simulink model "ARDroneHover_2020b"  (R2020b)
settings: Solver=ode1  StartTime=0.0  StopTime=inf  FixedStep=sampleTime  RelTol=1e-3  EnableMultiTasking=on
values from neighbouring files (symbols this model uses):
  sampleTime = 0.01    [setupHover.m]    (also in setupTT.m; setupWPTracking.m)
undefined symbols (not defined in the file or in its folder): DiscIntNeverNeededParam, Standard_Devices, UDP_Protocol
libraries: hdlsllib x6, dspnetwork x4, sldrtlib x3, simulink x1
(part 1 of 2)
settings Model: EnablePacing=on  ExtModeTrigDuration=100000  Creator=Paul  LastModifiedBy=dsor
settings SolverCC: AutoInsertRateTranBlk=on
settings DataIOCC: LimitDataPoints=on  SaveFormat=StructureWithTime  SignalLoggingSaveFormat=ModelDataLogs  ReturnWorkspaceOutputs=off  TimeSaveName=time
settings OptimizationCC: BlockReduction=off  OptimizeBlockIOStorage=off  BufferReuse=off  GlobalBufferReuse=off  ExpressionFolding=off  ExpressionDepthLimit=2147483647  LocalBlockOutputs=off  InitFltsAndDblsToZero=on  OptimizeDataStoreBuffers=off  BusAssignmentInplaceUpdate=off
settings DebuggingCC: UnderspecifiedInitializationDetection=Classic  MergeDetectMultiDrivingBlocksExec=none  SolverPrmCheckMsg=warning  FcnCallInpInsideContextMsg=warning  StateNameClashWarn=warning  SFUnexpectedBacktrackingDiag=warning  SFNoUnconditionalDefaultTransitionDiag=warning  SFExecutionAtInitializationDiag=none  ArithmeticOperatorsInVariantConditions=warning
settings ModelReferenceCC: PropagateSignalLabelsOutOfModel=off
settings SFSimCC: SimUseLocalCustomCode=off  CustomCodeUndefinedFunction=UseInterfaceOnly
settings RTWCC: Description=Simulink Desktop Real-Time  SystemTargetFile=sldrt.tlc  TemplateMakefile=sldrt.tmf  RTWUseLocalCustomCode=off  RTWCompilerOptimization=on
settings CodeAppCC: MaxIdLength=95  StateflowObjectComments=on
settings SimulinkDesktopRealTimeCC: TargetPreCompLibLocation=C:\Program Files\Polyspace\R2020b\toolbox\sldrt\lib\win64  TargetLangStandard=C89/C90 (ANSI)
settings ConfigComp: CovMetricSettings=dw  CovSaveCumulativeToWorkspaceVar=on  CovSaveSingleToWorkspaceVar=on  CovExternalEMLEnable=off

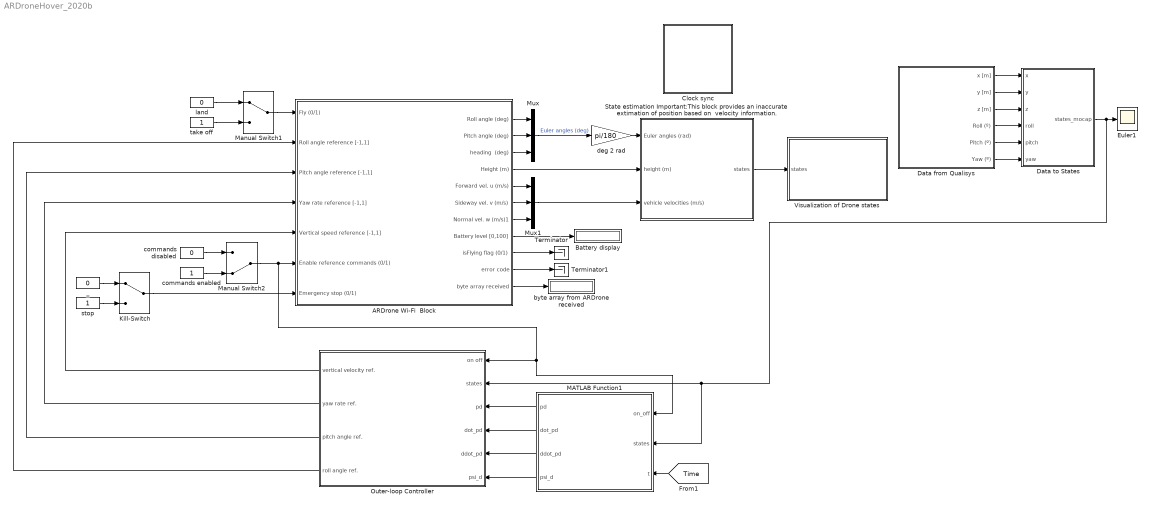
== system ARDroneHover_2020b ==
  ARDrone Wi-Fi  Block : Subsystem  AncestorBlock="ARBlocks/ARDrone Wi-Fi  Block"
  Battery display : Display
  Clock sync : Subsystem
  Data from Qualisys : Subsystem
  Data to States : Subsystem
  Euler1 : Scope
  Kill-Switch : ManualSwitch
  MATLAB Function1 : MATLAB Function  TreatAsAtomicUnit=on  SystemSampleTime=sampleTime
  Manual Switch1 : ManualSwitch
  Manual Switch2 : ManualSwitch  CurrentSetting=0
  Mux : Mux  Inputs=3
  Mux1 : Mux  Inputs=3
  Outer-loop Controller : Subsystem
  "State estimation Important:This block provides an inaccurate extimation of position based on  velocity information. " : Subsystem  AncestorBlock=|
      | ARBlocks/Position estimation
      | Important:This block provides an 
      | inaccurate extimation of position 
      | based on  velocity information.
  Terminator : Terminator
  Terminator1 : Terminator
  Visualization of Drone states : Subsystem
  _ : Constant  Value=0
  "byte array from ARDrone received " : Display
  commands disabled : Constant  Value=0
  commands enabled : Constant
  deg 2 rad : Gain  Gain=pi/180
  land : Constant  Value=0
  stop : Constant
  take off : Constant
  wires:
  _/1 -> Kill-Switch/1
  stop/1 -> Kill-Switch/2
  land/1 -> Manual Switch1/1
  take off/1 -> Manual Switch1/2
  commands disabled/1 -> Manual Switch2/1
  commands enabled/1 -> Manual Switch2/2
  Manual Switch1/1 -> ARDrone Wi-Fi  Block/1(Fly (0/1))
  Manual Switch2/1 -> ARDrone Wi-Fi  Block/6(Enable reference commands (0/1)), MATLAB Function1/1(on_off), Outer-loop Controller/1(on off)
  Kill-Switch/1 -> ARDrone Wi-Fi  Block/7(Emergency stop (0/1))
  ARDrone Wi-Fi  Block/1(Roll angle (deg)) -> Mux/1
  ARDrone Wi-Fi  Block/2(Pitch angle (deg)) -> Mux/2
  ARDrone Wi-Fi  Block/5(Forward vel. u (m/s)) -> Mux1/1
  ARDrone Wi-Fi  Block/6(Sideway vel. v (m/s)) -> Mux1/2
  ARDrone Wi-Fi  Block/7(Normal vel. w (m/s)1) -> Mux1/3
  Mux/1 -> deg 2 rad/1  "Euler angles (deg)"
  ARDrone Wi-Fi  Block/8(Battery level [0,100]) -> Battery display/1
  Outer-loop Controller/1(vertical velocity ref.) -> ARDrone Wi-Fi  Block/5(Vertical speed reference [-1,1])
  "State estimation Important:This block provides an inaccurate extimation of position based on  velocity information. "/1(states) -> Visualization of Drone states/1(states)
  deg 2 rad/1 -> "State estimation Important:This block provides an inaccurate extimation of position based on  velocity information. "/1(Euler angles (rad))
  Mux1/1 -> "State estimation Important:This block provides an inaccurate extimation of position based on  velocity information. "/3(vehicle velocities (m/s))
  ARDrone Wi-Fi  Block/3(heading  (deg)) -> Mux/3
  ARDrone Wi-Fi  Block/9(isFlying flag (0/1)) -> Terminator/1
  ARDrone Wi-Fi  Block/10(error code) -> Terminator1/1
  ARDrone Wi-Fi  Block/11(byte array received) -> "byte array from ARDrone received "/1
  Outer-loop Controller/2(yaw rate ref.) -> ARDrone Wi-Fi  Block/4(Yaw rate reference [-1,1])
  MATLAB Function1/2(dot_pd) -> Outer-loop Controller/4(dot_pd)
  MATLAB Function1/3(ddot_pd) -> Outer-loop Controller/5(ddot_pd)
  MATLAB Function1/4(psi_d) -> Outer-loop Controller/6(psi_d)
  MATLAB Function1/1(pd) -> Outer-loop Controller/3(pd)
  Data from Qualisys/1(x [m]) -> Data to States/1(x)
  Data from Qualisys/2(y [m]) -> Data to States/2(y)
  Data from Qualisys/3(z [m]) -> Data to States/3(z)
  Data from Qualisys/4(Roll (º)) -> Data to States/4(roll)
  Data from Qualisys/5(Pitch (º)) -> Data to States/5(pitch)
  Data from Qualisys/6(Yaw (º)) -> Data to States/6(yaw)
  [Time] -> MATLAB Function1/3(t)
  ARDrone Wi-Fi  Block/4(Height (m)) -> "State estimation Important:This block provides an inaccurate extimation of position based on  velocity information. "/2(height (m))
  Data to States/1(states_mocap) -> MATLAB Function1/2(states), Outer-loop Controller/2(states), Euler1/1
  Outer-loop Controller/4(roll angle ref.) -> ARDrone Wi-Fi  Block/2(Roll angle reference [-1,1])
  Outer-loop Controller/3(pitch angle ref.) -> ARDrone Wi-Fi  Block/3(Pitch angle reference [-1,1])

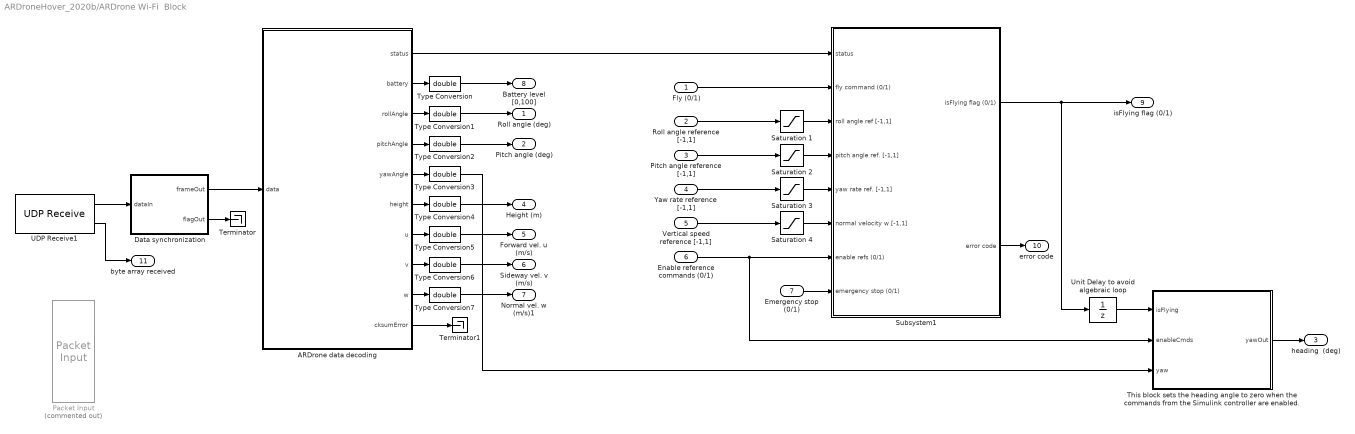
== system ARDroneHover_2020b/ARDrone Wi-Fi  Block ==
  Fly (0/1) : Inport
  Roll angle reference [-1,1] : Inport  Port=2
  Pitch angle reference [-1,1] : Inport  Port=3
  Yaw rate reference [-1,1] : Inport  Port=4
  Vertical speed reference [-1,1] : Inport  Port=5
  Enable reference commands (0/1) : Inport  Port=6
  Emergency stop (0/1) : Inport  Port=7
  ARDrone data decoding : MATLAB Function  TreatAsAtomicUnit=on
  "Data synchronization " : MATLAB Function  TreatAsAtomicUnit=on
  Packet Input : sldrtlib/Packet Input  Commented=on  SampleTime=sampleTime  MaxMissedTicks=100  ShowMissedTicks=off  YieldWhenWaiting=off  DrvName=Standard_Devices/UDP_Protocol  DrvAddress=5554  DrvOptions=[3232235777 5554]  PacketSize=500  DataTypes='500*uint8'  ShowReady=on  ShowError=off  PacketID=1  ByteOrder=1  ShowTimestamp=off
      settings: AttributesFormatString=UDP Protocol [5554]
  Saturation {1..4} (4 alike) : Saturate  UpperLimit=1  LowerLimit=-1
  Subsystem1 : Subsystem
  Terminator : Terminator
  Terminator1 : Terminator
  "This block sets the heading angle to zero when the commands from the Simulink controller are enabled. " : MATLAB Function  TreatAsAtomicUnit=on
  Type Conversion{,1..7} (8 alike) : DataTypeConversion  OutDataTypeStr=double
  UDP Receive1 : dspnetwork/UDP Receive  localURL='0.0.0.0'  localPort=5554  remoteURL='192.168.1.1'  remotePort=-1  recvBufferSize=500  dims=500  signalDatatype=uint8  isComplex=off  isVarSize=off  showBlockingTime=off  blockingTime=0  sampletime=sampleTime  blockPlatform=[]
  Unit Delay to avoid algebraic loop : UnitDelay  SampleTime=-1  HasFrameUpgradeWarning=on
  Roll angle (deg) : Outport  VectorParamsAs1DForOutWhenUnconnected=off
  Pitch angle (deg) : Outport  Port=2  VectorParamsAs1DForOutWhenUnconnected=off
  heading  (deg) : Outport  Port=3  VectorParamsAs1DForOutWhenUnconnected=off
  Height (m) : Outport  Port=4  VectorParamsAs1DForOutWhenUnconnected=off
  Forward vel. u (m/s) : Outport  Port=5  VectorParamsAs1DForOutWhenUnconnected=off
  Sideway vel. v (m/s) : Outport  Port=6  VectorParamsAs1DForOutWhenUnconnected=off
  Normal vel. w (m/s)1 : Outport  Port=7  VectorParamsAs1DForOutWhenUnconnected=off
  Battery level [0,100] : Outport  Port=8  VectorParamsAs1DForOutWhenUnconnected=off
  isFlying flag (0/1) : Outport  Port=9  VectorParamsAs1DForOutWhenUnconnected=off
  error code : Outport  Port=10  VectorParamsAs1DForOutWhenUnconnected=off
  byte array received : Outport  Port=11  VectorParamsAs1DForOutWhenUnconnected=off
  wires:
  Unit Delay to avoid algebraic loop/1 -> "This block sets the heading angle to zero when the commands from the Simulink controller are enabled. "/1(isFlying)
  "Data synchronization "/2(flagOut) -> Terminator/1
  Saturation 4/1 -> Subsystem1/6(normal velocity w [-1,1])
  Saturation 3/1 -> Subsystem1/5(yaw rate ref. [-1,1])
  Saturation 2/1 -> Subsystem1/4(pitch angle ref. [-1,1])
  Saturation 1/1 -> Subsystem1/3(roll angle ref [-1,1])
  Fly (0/1)/1 -> Subsystem1/2(fly command (0/1))
  "This block sets the heading angle to zero when the commands from the Simulink controller are enabled. "/1(yawOut) -> heading  (deg)/1
  Type Conversion3/1 -> "This block sets the heading angle to zero when the commands from the Simulink controller are enabled. "/3(yaw)
  Type Conversion7/1 -> Normal vel. w (m/s)1/1
  Type Conversion6/1 -> Sideway vel. v (m/s)/1
  Type Conversion5/1 -> Forward vel. u (m/s)/1
  Type Conversion4/1 -> Height (m)/1
  Type Conversion2/1 -> Pitch angle (deg)/1
  Type Conversion1/1 -> Roll angle (deg)/1
  Type Conversion/1 -> Battery level [0,100]/1
  ARDrone data decoding/10(cksumError) -> Terminator1/1
  Subsystem1/2(error code) -> error code/1
  Subsystem1/1(isFlying flag (0/1)) -> isFlying flag (0/1)/1, Unit Delay to avoid algebraic loop/1
  Emergency stop (0/1)/1 -> Subsystem1/8(emergency stop (0/1))
  Enable reference commands (0/1)/1 -> Subsystem1/7(enable refs (0/1)), "This block sets the heading angle to zero when the commands from the Simulink controller are enabled. "/2(enableCmds)
  Vertical speed reference [-1,1]/1 -> Saturation 4/1
  Yaw rate reference [-1,1]/1 -> Saturation 3/1
  Pitch angle reference [-1,1]/1 -> Saturation 2/1
  Roll angle reference [-1,1]/1 -> Saturation 1/1
  ARDrone data decoding/1(status) -> Subsystem1/1(status)
  UDP Receive1/2 -> byte array received/1
  ARDrone data decoding/9(w) -> Type Conversion7/1
  ARDrone data decoding/8(v) -> Type Conversion6/1
  ARDrone data decoding/7(u) -> Type Conversion5/1
  ARDrone data decoding/4(pitchAngle) -> Type Conversion2/1
  ARDrone data decoding/3(rollAngle) -> Type Conversion1/1
  ARDrone data decoding/6(height) -> Type Conversion4/1
  ARDrone data decoding/2(battery) -> Type Conversion/1
  ARDrone data decoding/5(yawAngle) -> Type Conversion3/1
  "Data synchronization "/1(frameOut) -> ARDrone data decoding/1(data)
  UDP Receive1/1 -> "Data synchronization "/1(dataIn)

== system ARDroneHover_2020b/Clock sync ==
  Clock1 : Clock
  To Workspace6 : ToWorkspace  VariableName=timeRT  SampleTime=sampleTime
  tag scope: Time=global
  wires:
  Clock1/1 -> [Time], To Workspace6/1

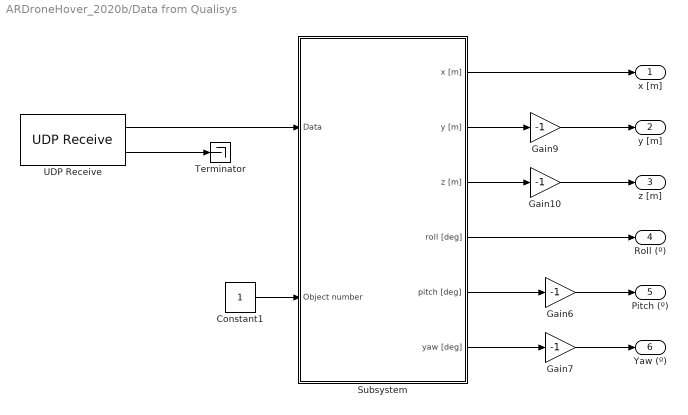
== system ARDroneHover_2020b/Data from Qualisys ==
  Constant1 : Constant
  Gain{6..7,9..10} (4 alike) : Gain  Gain=-1
  Subsystem : Subsystem
  Terminator : Terminator
  UDP Receive : dspnetwork/UDP Receive  localURL='0.0.0.0'  localPort=9089  remoteURL='169.254.54.40'  remotePort=-1  recvBufferSize=64  dims=255  signalDatatype=uint8  isComplex=off  isVarSize=off  showBlockingTime=off  blockingTime=0  sampletime=sampleTime  blockPlatform=[]
  x [m] : Outport
  y [m] : Outport  Port=2
  z [m] : Outport  Port=3
  Roll (º) : Outport  Port=4
  Pitch (º) : Outport  Port=5
  Yaw (º) : Outport  Port=6
  wires:
  Subsystem/3(z [m]) -> Gain10/1
  Subsystem/2(y [m]) -> Gain9/1
  Constant1/1 -> Subsystem/2(Object number)
  Subsystem/5(pitch [deg]) -> Gain6/1
  Gain7/1 -> Yaw (º)/1
  Gain10/1 -> z [m]/1
  Gain6/1 -> Pitch (º)/1
  Gain9/1 -> y [m]/1
  Subsystem/1(x [m]) -> x [m]/1
  UDP Receive/2 -> Terminator/1
  UDP Receive/1 -> Subsystem/1(Data)
  Subsystem/4(roll [deg]) -> Roll (º)/1
  Subsystem/6(yaw [deg]) -> Gain7/1

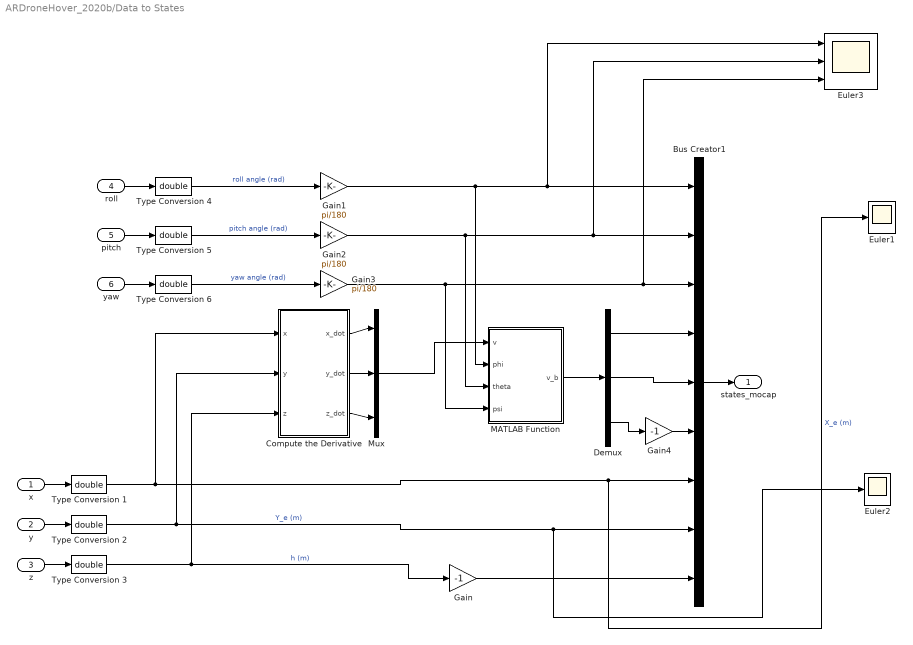
== system ARDroneHover_2020b/Data to States ==
  x : Inport
  y : Inport  Port=2
  z : Inport  Port=3
  roll : Inport  Port=4
  pitch : Inport  Port=5
  yaw : Inport  Port=6
  Bus Creator1 : BusCreator  Inputs=9
  Compute the Derivative : Subsystem
  Demux : Demux  Outputs=3
  Euler1 : Scope
  Euler2 : Scope
  Euler3 : Scope  NumInputPorts=3
  Gain : Gain  Gain=-1
  Gain1 : Gain  Gain=pi/180
  Gain2 : Gain  Gain=pi/180
  Gain3 : Gain  Gain=pi/180
  Gain4 : Gain  Gain=-1
  MATLAB Function : MATLAB Function  TreatAsAtomicUnit=on
  Mux : Mux  Inputs=3
  Type Conversion {1..6} (6 alike) : DataTypeConversion  OutDataTypeStr=double
  states_mocap : Outport  VectorParamsAs1DForOutWhenUnconnected=off
  wires:
  x/1 -> Type Conversion 1/1
  y/1 -> Type Conversion 2/1
  z/1 -> Type Conversion 3/1
  roll/1 -> Type Conversion 4/1
  pitch/1 -> Type Conversion 5/1
  yaw/1 -> Type Conversion 6/1
  Type Conversion 6/1 -> Gain3/1  "yaw angle (rad)"
  Type Conversion 4/1 -> Gain1/1  "roll angle (rad)"
  Type Conversion 5/1 -> Gain2/1  "pitch angle (rad)"
  Type Conversion 1/1 -> Compute the Derivative/1(x), Euler1/1, Bus Creator1/7  "X_e (m)"
  Type Conversion 3/1 -> Compute the Derivative/3(z), Gain/1  "h (m)"
  Type Conversion 2/1 -> Compute the Derivative/2(y), Euler2/1, Bus Creator1/8  "Y_e (m)"
  Gain/1 -> Bus Creator1/9
  Compute the Derivative/1(x_dot) -> Mux/1
  Compute the Derivative/2(y_dot) -> Mux/2
  Compute the Derivative/3(z_dot) -> Mux/3
  MATLAB Function/1(v_b) -> Demux/1
  Mux/1 -> MATLAB Function/1(v)
  Gain1/1 -> Euler3/1, Bus Creator1/1, MATLAB Function/2(phi)
  Gain2/1 -> MATLAB Function/3(theta), Euler3/2, Bus Creator1/2
  Gain3/1 -> MATLAB Function/4(psi), Euler3/3, Bus Creator1/3
  Demux/1 -> Bus Creator1/4
  Demux/2 -> Bus Creator1/5
  Gain4/1 -> Bus Creator1/6
  Demux/3 -> Gain4/1
  Bus Creator1/1 -> states_mocap/1

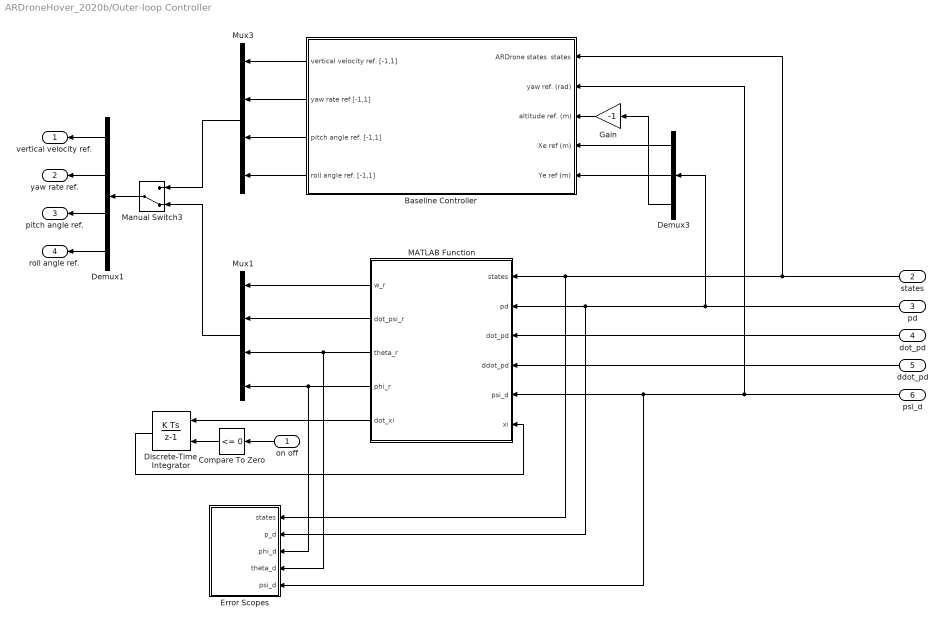
== system ARDroneHover_2020b/Outer-loop Controller ==
  on off : Inport  PortDimensions=1
  states : Inport  Port=2
  pd : Inport  Port=3  PortDimensions=[3 1]
  dot_pd : Inport  Port=4  PortDimensions=[3 1]
  ddot_pd : Inport  Port=5  PortDimensions=[3 1]
  psi_d : Inport  Port=6  PortDimensions=1
  Baseline Controller : Subsystem  AncestorBlock=ARBlocks/Baseline Controller
  Compare To Zero : simulink/Logic and Bit Operations/Compare To Zero  relop=<=  OutDataTypeStr=boolean
  Demux1 : Demux  Outputs=[1,1,1,1]
  Demux3 : Demux  Outputs=[1,1,1]
  Discrete-Time Integrator : DiscreteIntegrator  ExternalReset=level  InitialCondition=[0;0;0;0]  SampleTime=sampleTime  LimitOutput=on  UpperSaturationLimit=100  LowerSaturationLimit=-100  ICPrevOutput=DiscIntNeverNeededParam  ICPrevScaledInput=DiscIntNeverNeededParam
  Error Scopes : Subsystem
  Gain : Gain  Gain=-1
  MATLAB Function : MATLAB Function  TreatAsAtomicUnit=on  SystemSampleTime=sampleTime
  Manual Switch3 : ManualSwitch  CurrentSetting=0
  Mux1 : Mux  Inputs=[1,1,1,1]
  Mux3 : Mux  Inputs=[1,1,1,1]
  vertical velocity ref. : Outport  VectorParamsAs1DForOutWhenUnconnected=off
  yaw rate ref. : Outport  Port=2  VectorParamsAs1DForOutWhenUnconnected=off
  pitch angle ref. : Outport  Port=3  VectorParamsAs1DForOutWhenUnconnected=off
  roll angle ref. : Outport  Port=4  VectorParamsAs1DForOutWhenUnconnected=off
  wires:
  states/1 -> MATLAB Function/1(states), Error Scopes/1(states), Baseline Controller/1("ARDrone states  states ")
  MATLAB Function/1(w_r) -> Mux1/1
  MATLAB Function/3(theta_r) -> Error Scopes/4(theta_d), Mux1/3
  MATLAB Function/4(phi_r) -> Mux1/4, Error Scopes/3(phi_d)
  MATLAB Function/2(dot_psi_r) -> Mux1/2
  MATLAB Function/5(dot_xi) -> Discrete-Time Integrator/1
  Discrete-Time Integrator/1 -> MATLAB Function/6(xi)
  pd/1 -> Demux3/1, MATLAB Function/2(pd), Error Scopes/2(p_d)
  dot_pd/1 -> MATLAB Function/3(dot_pd)
  ddot_pd/1 -> MATLAB Function/4(ddot_pd)
  psi_d/1 -> Baseline Controller/2(yaw ref. (rad)), MATLAB Function/5(psi_d), Error Scopes/5(psi_d)
  Demux3/1 -> Baseline Controller/4(Xe ref (m))
  Demux3/2 -> Baseline Controller/5(Ye ref (m))
  Demux3/3 -> Gain/1
  Baseline Controller/4(roll angle ref. [-1,1]) -> Mux3/4
  Baseline Controller/3(pitch angle ref. [-1,1]) -> Mux3/3
  Baseline Controller/2(yaw rate ref [-1,1]) -> Mux3/2
  Baseline Controller/1(vertical velocity ref. [-1,1]) -> Mux3/1
  Mux3/1 -> Manual Switch3/1
  Demux1/1 -> vertical velocity ref./1
  Demux1/2 -> yaw rate ref./1
  Demux1/3 -> pitch angle ref./1
  Demux1/4 -> roll angle ref./1
  Manual Switch3/1 -> Demux1/1
  Mux1/1 -> Manual Switch3/2
  on off/1 -> Compare To Zero/1
  Compare To Zero/1 -> Discrete-Time Integrator/2
  Gain/1 -> Baseline Controller/3(altitude ref. (m))

== system ARDroneHover_2020b/State estimation Important:This block provides an inaccurate extimation of position based on  velocity information.  ==
  Euler angles (rad) : Inport
  height (m) : Inport  Port=2
  vehicle velocities (m/s) : Inport  Port=3
  Bus Creator1 : BusCreator  Inputs=9
  Demux : Demux  Outputs=3
  Demux1 : Demux  Outputs=3
  Demux2 : Demux  Outputs=3
  Position estimation : Subsystem
  states : Outport  VectorParamsAs1DForOutWhenUnconnected=off
  wires:
  height (m)/1 -> Position estimation/2(height (m))
  Bus Creator1/1 -> states/1
  Demux2/3 -> Bus Creator1/9  "h (m)"
  Demux2/2 -> Bus Creator1/8  "Y_e (m)"
  Demux2/1 -> Bus Creator1/7  "X_e (m)"
  Demux1/3 -> Bus Creator1/6  "vertical velocity - h_dot (m/s)"
  Demux1/2 -> Bus Creator1/5  "sideward velocity - v (m/s)"
  Demux1/1 -> Bus Creator1/4  "forward velocity- u (m/s)"
  Demux/3 -> Bus Creator1/3  "yaw angle (rad)"
  Demux/2 -> Bus Creator1/2  "pitch angle (rad)"
  Demux/1 -> Bus Creator1/1  "roll angle (rad)"
  Position estimation/1(Inertial position Xe,Ye,h (m)) -> Demux2/1
  Euler angles (rad)/1 -> Demux/1, Position estimation/1(Vehicle euler angles (rad))
  vehicle velocities (m/s)/1 -> Position estimation/3(vehicle frame velocities (m/s)), Demux1/1

== system ARDroneHover_2020b/Visualization of Drone states ==
  states : Inport
  Bus Selector2 : BusSelector  OutputSignals=yaw angle (rad),X_e (m),Y_e (m),h (m)
  Height (m) : Scope
  Inertial position along Xe (m) : Scope
  Inertial position along Ye (m) : Scope
  To Workspace : ToWorkspace  VariableName=states  SaveFormat=Structure With Time  SampleTime=-1
  deg 2 rad1 : Gain  Gain=180/pi
  heading (deg) : Scope
  wires:
  states/1 -> To Workspace/1, Bus Selector2/1
  Bus Selector2/1 -> deg 2 rad1/1  "<yaw angle (rad)>"
  Bus Selector2/2 -> Inertial position along Xe (m)/1  "<X_e (m)>"
  Bus Selector2/3 -> Inertial position along Ye (m)/1  "<Y_e (m)>"
  Bus Selector2/4 -> Height (m)/1  "<h (m)>"
  deg 2 rad1/1 -> heading (deg)/1

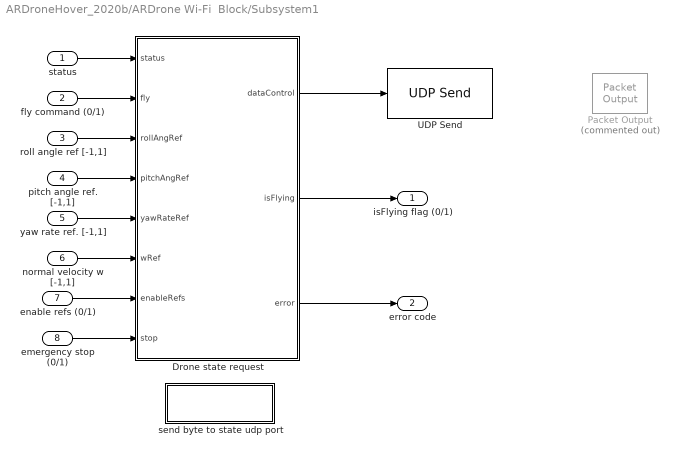
== system ARDroneHover_2020b/ARDrone Wi-Fi  Block/Subsystem1 ==
  status : Inport
  fly command (0/1) : Inport  Port=2
  roll angle ref [-1,1] : Inport  Port=3
  pitch angle ref. [-1,1] : Inport  Port=4
  yaw rate ref. [-1,1] : Inport  Port=5
  normal velocity w [-1,1] : Inport  Port=6
  enable refs (0/1) : Inport  Port=7
  emergency stop (0/1) : Inport  Port=8
  Drone state request : MATLAB Function  TreatAsAtomicUnit=on  SystemSampleTime=sampleTime
  Packet Output : sldrtlib/Packet Output  Commented=on  SampleTime=sampleTime*7  MaxMissedTicks=100  ShowMissedTicks=off  YieldWhenWaiting=off  DrvName=Standard_Devices/UDP_Protocol  DrvAddress=5556  DrvOptions=[3232235777 5556]  PacketSize=150  DataTypes='150*uint8'  ShowReady=off  ShowError=off  PacketID=1  ByteOrder=1  InitialValue=[]  FinalValue=[]
      settings: AttributesFormatString=UDP Protocol [5556]
  UDP Send : dspnetwork/UDP Send  remoteURL='192.168.1.1'  remotePort=5556  localURL='0.0.0.0'  localPortSource=Specify via dialog  localPort=5556  sendBufferSize=8192  sampletime=-1  blockPlatform=[]  separateLengthPort=0
  "send byte to state udp port " : Subsystem
  isFlying flag (0/1) : Outport  VectorParamsAs1DForOutWhenUnconnected=off
  error code : Outport  Port=2  VectorParamsAs1DForOutWhenUnconnected=off
  wires:
  Drone state request/3(error) -> error code/1
  emergency stop (0/1)/1 -> Drone state request/8(stop)
  enable refs (0/1)/1 -> Drone state request/7(enableRefs)
  normal velocity w [-1,1]/1 -> Drone state request/6(wRef)
  yaw rate ref. [-1,1]/1 -> Drone state request/5(yawRateRef)
  roll angle ref [-1,1]/1 -> Drone state request/3(rollAngRef)
  Drone state request/2(isFlying) -> isFlying flag (0/1)/1
  status/1 -> Drone state request/1(status)
  pitch angle ref. [-1,1]/1 -> Drone state request/4(pitchAngRef)
  fly command (0/1)/1 -> Drone state request/2(fly)
  Drone state request/1(dataControl) -> UDP Send/1

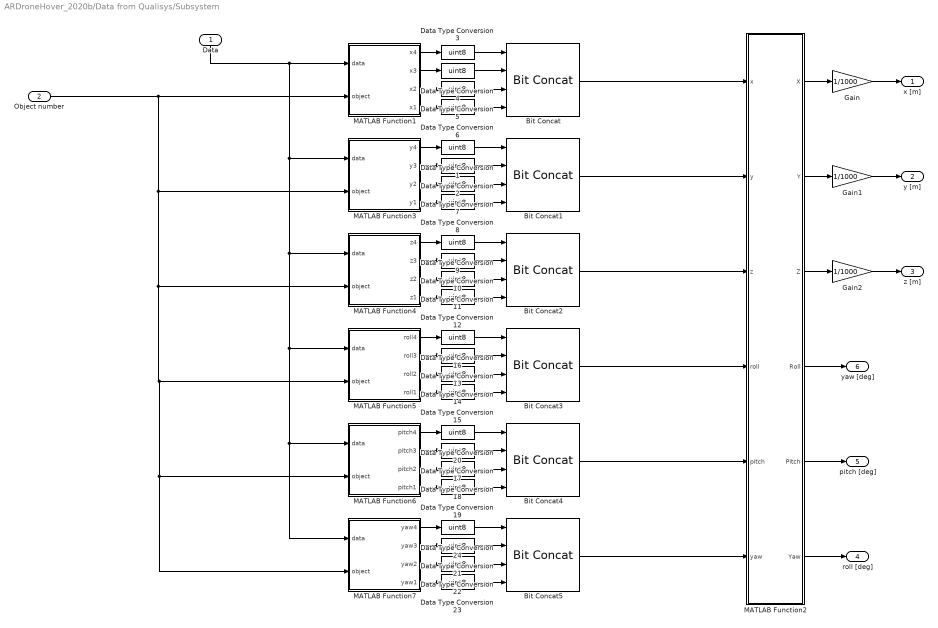
== system ARDroneHover_2020b/Data from Qualisys/Subsystem ==
  Data : Inport
  Object number : Inport  Port=2
  Bit Concat{,1..5} (6 alike) : hdlsllib/Logic and Bit Operations/Bit Concat  numInputs=4
  Data Type Conversion{1..24} (24 alike) : DataTypeConversion  OutDataTypeStr=uint8
  Gain : Gain  Gain=1/1000
  Gain1 : Gain  Gain=1/1000
  Gain2 : Gain  Gain=1/1000
  MATLAB Function1 : MATLAB Function  TreatAsAtomicUnit=on
  MATLAB Function2 : MATLAB Function  TreatAsAtomicUnit=on
  MATLAB Function3 : MATLAB Function  TreatAsAtomicUnit=on
  MATLAB Function4 : MATLAB Function  TreatAsAtomicUnit=on
  MATLAB Function5 : MATLAB Function  TreatAsAtomicUnit=on
  MATLAB Function6 : MATLAB Function  TreatAsAtomicUnit=on
  MATLAB Function7 : MATLAB Function  TreatAsAtomicUnit=on
  x [m] : Outport  VectorParamsAs1DForOutWhenUnconnected=off
  y [m] : Outport  Port=2  VectorParamsAs1DForOutWhenUnconnected=off
  z [m] : Outport  Port=3  VectorParamsAs1DForOutWhenUnconnected=off
  roll [deg] : Outport  Port=4  VectorParamsAs1DForOutWhenUnconnected=off
  pitch [deg] : Outport  Port=5  VectorParamsAs1DForOutWhenUnconnected=off
  yaw [deg] : Outport  Port=6  VectorParamsAs1DForOutWhenUnconnected=off
  wires:
  Data Type Conversion6/1 -> Bit Concat/4
  Data Type Conversion3/1 -> Bit Concat/1
  MATLAB Function1/3(x2) -> Data Type Conversion5/1
  MATLAB Function2/1(X) -> Gain/1
  MATLAB Function4/1(z4) -> Data Type Conversion9/1
  MATLAB Function4/2(z3) -> Data Type Conversion10/1
  Bit Concat2/1 -> MATLAB Function2/3(z)
  Data Type Conversion12/1 -> Bit Concat2/4
  Data Type Conversion11/1 -> Bit Concat2/3
  MATLAB Function4/4(z1) -> Data Type Conversion12/1
  Data Type Conversion10/1 -> Bit Concat2/2
  MATLAB Function4/3(z2) -> Data Type Conversion11/1
  Data Type Conversion9/1 -> Bit Concat2/1
  MATLAB Function2/5(Pitch) -> pitch [deg]/1
  MATLAB Function2/2(Y) -> Gain1/1
  MATLAB Function2/6(Yaw) -> roll [deg]/1
  Data Type Conversion14/1 -> Bit Concat3/3
  MATLAB Function5/3(roll2) -> Data Type Conversion14/1
  Bit Concat3/1 -> MATLAB Function2/4(roll)
  MATLAB Function5/2(roll3) -> Data Type Conversion13/1
  Data Type Conversion13/1 -> Bit Concat3/2
  Data Type Conversion15/1 -> Bit Concat3/4
  Data Type Conversion16/1 -> Bit Concat3/1
  MATLAB Function5/1(roll4) -> Data Type Conversion16/1
  MATLAB Function5/4(roll1) -> Data Type Conversion15/1
  MATLAB Function1/2(x3) -> Data Type Conversion4/1
  MATLAB Function1/4(x1) -> Data Type Conversion6/1
  MATLAB Function1/1(x4) -> Data Type Conversion3/1
  Bit Concat/1 -> MATLAB Function2/1(x)
  MATLAB Function2/3(Z) -> Gain2/1
  MATLAB Function2/4(Roll) -> yaw [deg]/1
  Data Type Conversion5/1 -> Bit Concat/3
  Data/1 -> MATLAB Function1/1(data), MATLAB Function7/1(data), MATLAB Function6/1(data), MATLAB Function5/1(data), MATLAB Function4/1(data), MATLAB Function3/1(data)
  Data Type Conversion4/1 -> Bit Concat/2
  Data Type Conversion20/1 -> Bit Concat4/1
  MATLAB Function6/2(pitch3) -> Data Type Conversion17/1
  MATLAB Function6/3(pitch2) -> Data Type Conversion18/1
  Data Type Conversion17/1 -> Bit Concat4/2
  MATLAB Function6/1(pitch4) -> Data Type Conversion20/1
  Data Type Conversion19/1 -> Bit Concat4/4
  MATLAB Function6/4(pitch1) -> Data Type Conversion19/1
  Bit Concat4/1 -> MATLAB Function2/5(pitch)
  Data Type Conversion18/1 -> Bit Concat4/3
  MATLAB Function7/1(yaw4) -> Data Type Conversion24/1
  Bit Concat5/1 -> MATLAB Function2/6(yaw)
  Data Type Conversion24/1 -> Bit Concat5/1
  Data Type Conversion22/1 -> Bit Concat5/3
  MATLAB Function7/3(yaw2) -> Data Type Conversion22/1
  Data Type Conversion21/1 -> Bit Concat5/2
  Object number/1 -> MATLAB Function1/2(object), MATLAB Function7/2(object), MATLAB Function6/2(object), MATLAB Function5/2(object), MATLAB Function4/2(object), MATLAB Function3/2(object)
  MATLAB Function7/4(yaw1) -> Data Type Conversion23/1
  Data Type Conversion23/1 -> Bit Concat5/4
  MATLAB Function7/2(yaw3) -> Data Type Conversion21/1
  MATLAB Function3/1(y4) -> Data Type Conversion1/1
  MATLAB Function3/3(y2) -> Data Type Conversion7/1
  Data Type Conversion8/1 -> Bit Concat1/4
  Data Type Conversion2/1 -> Bit Concat1/2
  MATLAB Function3/4(y1) -> Data Type Conversion8/1
  MATLAB Function3/2(y3) -> Data Type Conversion2/1
  Data Type Conversion1/1 -> Bit Concat1/1
  Bit Concat1/1 -> MATLAB Function2/2(y)
  Data Type Conversion7/1 -> Bit Concat1/3
  Gain/1 -> x [m]/1
  Gain1/1 -> y [m]/1
  Gain2/1 -> z [m]/1

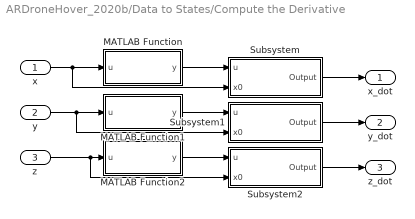
== system ARDroneHover_2020b/Data to States/Compute the Derivative ==
  x : Inport
  y : Inport  Port=2
  z : Inport  Port=3
  MATLAB Function : MATLAB Function  TreatAsAtomicUnit=on
  MATLAB Function1 : MATLAB Function  TreatAsAtomicUnit=on
  MATLAB Function2 : MATLAB Function  TreatAsAtomicUnit=on
  Subsystem : Subsystem
  Subsystem1 : Subsystem
  Subsystem2 : Subsystem
  x_dot : Outport  VectorParamsAs1DForOutWhenUnconnected=off
  y_dot : Outport  Port=2  VectorParamsAs1DForOutWhenUnconnected=off
  z_dot : Outport  Port=3  VectorParamsAs1DForOutWhenUnconnected=off
  wires:
  x/1 -> Subsystem/2(x0), MATLAB Function/1(u)
  z/1 -> Subsystem2/2(x0), MATLAB Function2/1(u)
  y/1 -> Subsystem1/2(x0), MATLAB Function1/1(u)
  MATLAB Function/1(y) -> Subsystem/1(u)
  Subsystem/1(Output) -> x_dot/1
  MATLAB Function1/1(y) -> Subsystem1/1(u)
  Subsystem1/1(Output) -> y_dot/1
  MATLAB Function2/1(y) -> Subsystem2/1(u)
  Subsystem2/1(Output) -> z_dot/1

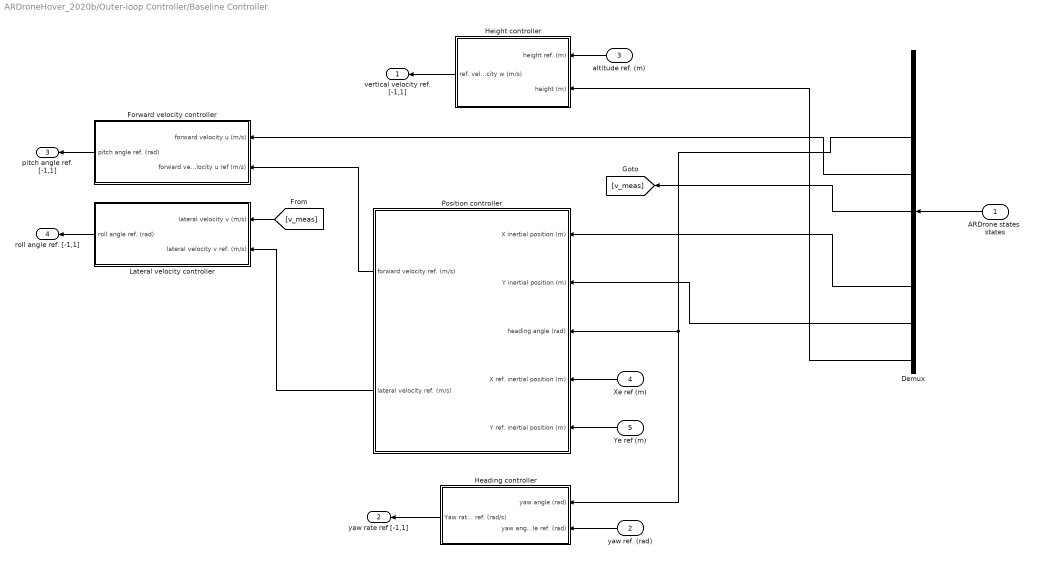
== system ARDroneHover_2020b/Outer-loop Controller/Baseline Controller ==
  "ARDrone states  states " : Inport
  yaw ref. (rad) : Inport  Port=2
  altitude ref. (m) : Inport  Port=3
  Xe ref (m) : Inport  Port=4
  Ye ref (m) : Inport  Port=5
  Demux : Demux  Outputs=9
  "Forward velocity controller " : Subsystem
  Heading controller : Subsystem
  "Height controller " : Subsystem
  Lateral velocity controller : Subsystem
  Position controller : Subsystem
  vertical velocity ref. [-1,1] : Outport  VectorParamsAs1DForOutWhenUnconnected=off
  yaw rate ref [-1,1] : Outport  Port=2  VectorParamsAs1DForOutWhenUnconnected=off
  pitch angle ref. [-1,1] : Outport  Port=3  VectorParamsAs1DForOutWhenUnconnected=off
  roll angle ref. [-1,1] : Outport  Port=4  VectorParamsAs1DForOutWhenUnconnected=off
  wires:
  [v_meas] -> Lateral velocity controller/1(lateral velocity v (m/s))
  Demux/5 -> [v_meas]
  Position controller/2(lateral velocity ref. (m/s)) -> Lateral velocity controller/2(lateral velocity v ref. (m/s))
  Position controller/1(forward velocity ref. (m/s)) -> "Forward velocity controller "/2(forward velocity u ref (m/s))
  Ye ref (m)/1 -> Position controller/5(Y ref. inertial position (m))
  Xe ref (m)/1 -> Position controller/4(X ref. inertial position (m))
  Demux/8 -> Position controller/2(Y inertial position (m))
  Demux/7 -> Position controller/1(X inertial position (m))
  Heading controller/1(Yaw rate ref. (rad/s)) -> yaw rate ref [-1,1]/1
  yaw ref. (rad)/1 -> Heading controller/2(yaw angle ref. (rad))
  "Forward velocity controller "/1(pitch angle ref. (rad)) -> pitch angle ref. [-1,1]/1
  Demux/4 -> "Forward velocity controller "/1(forward velocity u (m/s))
  Lateral velocity controller/1(roll angle ref. (rad)) -> roll angle ref. [-1,1]/1
  "Height controller "/1(ref. velocity w (m/s)) -> vertical velocity ref. [-1,1]/1
  Demux/9 -> "Height controller "/2(height (m))
  altitude ref. (m)/1 -> "Height controller "/1(height ref. (m))
  Demux/3 -> Position controller/3(heading angle (rad)), Heading controller/1(yaw angle (rad))
  "ARDrone states  states "/1 -> Demux/1

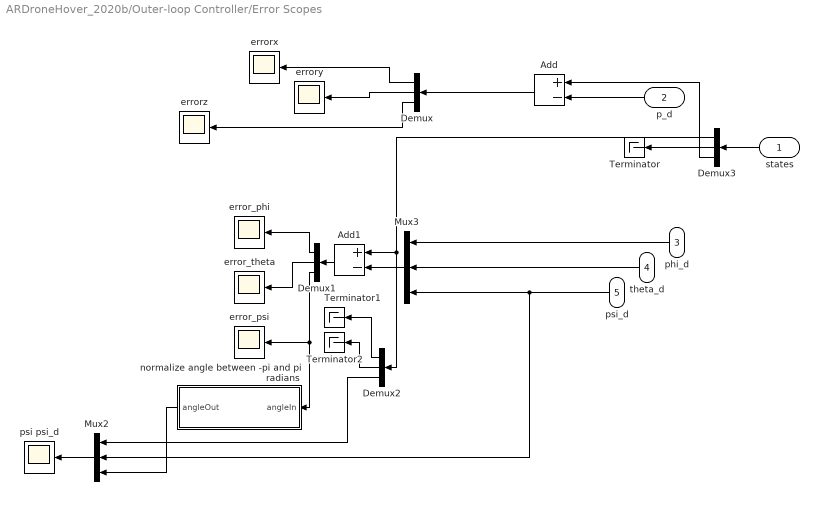
== system ARDroneHover_2020b/Outer-loop Controller/Error Scopes ==
  states : Inport
  p_d : Inport  Port=2
  phi_d : Inport  Port=3
  theta_d : Inport  Port=4
  psi_d : Inport  Port=5
  Add : Sum  Inputs=+-
  Add1 : Sum  Inputs=+-
  Demux : Demux  Outputs=3
  Demux1 : Demux  Outputs=[1,1,1]
  Demux2 : Demux  Outputs=[1,1,1]
  Demux3 : Demux  Outputs=[3,3,3]
  Mux2 : Mux  Inputs=[1,1,1]
  Mux3 : Mux  Inputs=[1,1,1]
  Terminator : Terminator
  Terminator1 : Terminator
  Terminator2 : Terminator
  error_phi : Scope
  error_psi : Scope
  error_theta : Scope
  errorx : Scope
  errory : Scope
  errorz : Scope
  normalize angle between -pi and pi radians : MATLAB Function  TreatAsAtomicUnit=on
  psi psi_d : Scope
  wires:
  Add/1 -> Demux/1
  Demux/1 -> errorx/1
  Demux/3 -> errorz/1
  Demux/2 -> errory/1
  Demux1/1 -> error_phi/1
  Demux1/2 -> error_theta/1
  p_d/1 -> Add/2
  phi_d/1 -> Mux3/1
  theta_d/1 -> Mux3/2
  psi_d/1 -> Mux2/2, Mux3/3
  Mux2/1 -> psi psi_d/1
  Demux1/3 -> normalize angle between -pi and pi radians/1(angleIn), error_psi/1
  Demux2/3 -> Mux2/1
  normalize angle between -pi and pi radians/1(angleOut) -> Mux2/3
  states/1 -> Demux3/1
  Demux3/3 -> Add/1
  Demux3/1 -> Add1/1, Demux2/1
  Add1/1 -> Demux1/1
  Mux3/1 -> Add1/2
  Demux3/2 -> Terminator/1
  Demux2/1 -> Terminator1/1
  Demux2/2 -> Terminator2/1

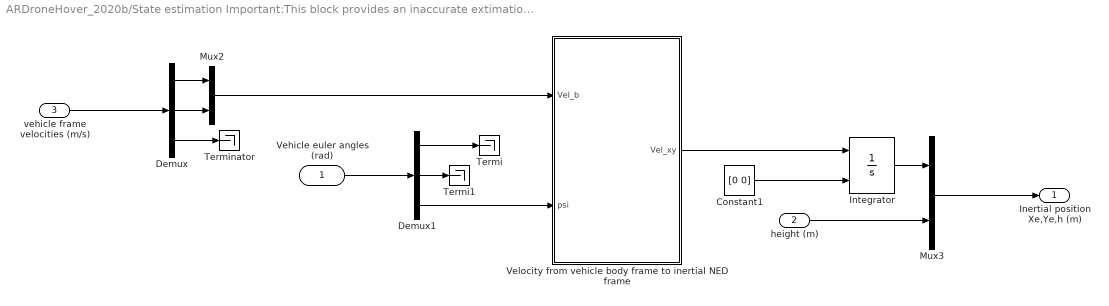
== system ARDroneHover_2020b/State estimation Important:This block provides an inaccurate extimation of position based on  velocity information. /Position estimation ==
  Vehicle euler angles (rad) : Inport
  height (m) : Inport  Port=2
  vehicle frame velocities (m/s) : Inport  Port=3
  Constant1 : Constant  Value=[0 0]
  Demux : Demux  Outputs=3
  Demux1 : Demux  Outputs=3
  Integrator : Integrator  InitialConditionSource=external
  Mux2 : Mux  Inputs=2
  Mux3 : Mux  Inputs=2
  Termi : Terminator
  Termi1 : Terminator
  Terminator : Terminator
  Velocity from vehicle body frame to inertial NED  frame : MATLAB Function  TreatAsAtomicUnit=on
  Inertial position Xe,Ye,h (m) : Outport  VectorParamsAs1DForOutWhenUnconnected=off
  wires:
  Mux3/1 -> Inertial position Xe,Ye,h (m)/1
  height (m)/1 -> Mux3/2
  Vehicle euler angles (rad)/1 -> Demux1/1
  vehicle frame velocities (m/s)/1 -> Demux/1
  Demux1/3 -> Velocity from vehicle body frame to inertial NED  frame/2(psi)
  Integrator/1 -> Mux3/1
  Constant1/1 -> Integrator/2
  Velocity from vehicle body frame to inertial NED  frame/1(Vel_xy) -> Integrator/1
  Demux1/2 -> Termi1/1
  Demux1/1 -> Termi/1
  Mux2/1 -> Velocity from vehicle body frame to inertial NED  frame/1(Vel_b)
  Demux/1 -> Mux2/1
  Demux/2 -> Mux2/2
  Demux/3 -> Terminator/1

== system ARDroneHover_2020b/ARDrone Wi-Fi  Block/Subsystem1/send byte to state udp port  ==
  Constant : Constant  Value=[1 ;13]  OutDataTypeStr=uint8
  Packet Output : sldrtlib/Packet Output  Commented=on  SampleTime=sampleTime*10  MaxMissedTicks=100  ShowMissedTicks=off  YieldWhenWaiting=off  DrvName=Standard_Devices/UDP_Protocol  DrvAddress=5554  DrvOptions=[3232235777 5554]  PacketSize=2  DataTypes='2*uint8'  ShowReady=off  ShowError=off  PacketID=1  ByteOrder=1  InitialValue=[]  FinalValue=[]
      settings: AttributesFormatString=UDP Protocol [5554]
  Rate Transition : RateTransition
  UDP Send : dspnetwork/UDP Send  remoteURL='192.168.1.1'  remotePort=5554  localURL='0.0.0.0'  localPortSource=Specify via dialog  localPort=5554  sendBufferSize=8192  sampletime=-1  blockPlatform=[]  separateLengthPort=0
  wires:
  Constant/1 -> Rate Transition/1
  Rate Transition/1 -> UDP Send/1

== system ARDroneHover_2020b/Data to States/Compute the Derivative/Subsystem ==
  u : Inport
  x0 : Inport  Port=2
  Gain : Gain  Gain=6
  Integrator : Integrator  InitialConditionSource=external
  Sum : Sum  Inputs=|+-
  Output : Outport  VectorParamsAs1DForOutWhenUnconnected=off
  wires:
  Integrator/1 -> Sum/2
  u/1 -> Sum/1
  Gain/1 -> Output/1, Integrator/1
  Sum/1 -> Gain/1
  x0/1 -> Integrator/2

== system ARDroneHover_2020b/Data to States/Compute the Derivative/Subsystem1 ==
  u : Inport
  x0 : Inport  Port=2
  Gain : Gain  Gain=6
  Integrator : Integrator  InitialConditionSource=external
  Sum : Sum  Inputs=|+-
  Output : Outport  VectorParamsAs1DForOutWhenUnconnected=off
  wires:
  Integrator/1 -> Sum/2
  u/1 -> Sum/1
  Gain/1 -> Output/1, Integrator/1
  Sum/1 -> Gain/1
  x0/1 -> Integrator/2

== system ARDroneHover_2020b/Data to States/Compute the Derivative/Subsystem2 ==
  u : Inport
  x0 : Inport  Port=2
  Gain : Gain  Gain=6
  Integrator : Integrator  InitialConditionSource=external
  Sum : Sum  Inputs=|+-
  Output : Outport  VectorParamsAs1DForOutWhenUnconnected=off
  wires:
  Integrator/1 -> Sum/2
  u/1 -> Sum/1
  Gain/1 -> Output/1, Integrator/1
  Sum/1 -> Gain/1
  x0/1 -> Integrator/2

== system ARDroneHover_2020b/Outer-loop Controller/Baseline Controller/Forward velocity controller  ==
  forward velocity u (m/s) : Inport
  forward velocity u ref (m/s) : Inport  Port=2
  Gain : Gain  Gain=-0.5*1/2
  Sum2 : Sum  Inputs=|-+
  pitch angle ref. (rad) : Outport  VectorParamsAs1DForOutWhenUnconnected=off
  wires:
  forward velocity u ref (m/s)/1 -> Sum2/2
  Gain/1 -> pitch angle ref. (rad)/1
  Sum2/1 -> Gain/1
  forward velocity u (m/s)/1 -> Sum2/1

== system ARDroneHover_2020b/Outer-loop Controller/Baseline Controller/Heading controller ==
  yaw angle (rad) : Inport
  yaw angle ref. (rad) : Inport  Port=2
  Sum1 : Sum  Inputs=|-+
  normalize angle between -pi and pi radians : MATLAB Function  TreatAsAtomicUnit=on
  proportional control gain - yaw : Gain  Gain=1.5
  Yaw rate ref. (rad/s) : Outport  VectorParamsAs1DForOutWhenUnconnected=off
  wires:
  yaw angle ref. (rad)/1 -> Sum1/2
  proportional control gain - yaw/1 -> Yaw rate ref. (rad/s)/1
  yaw angle (rad)/1 -> Sum1/1
  normalize angle between -pi and pi radians/1(angleOut) -> proportional control gain - yaw/1
  Sum1/1 -> normalize angle between -pi and pi radians/1(angleIn)

== system ARDroneHover_2020b/Outer-loop Controller/Baseline Controller/Height controller  ==
  height ref. (m) : Inport
  height (m) : Inport  Port=2
  Sum3 : Sum  Inputs=|-+
  proportional control gain : Gain
  ref. velocity w (m/s) : Outport  VectorParamsAs1DForOutWhenUnconnected=off
  wires:
  height ref. (m)/1 -> Sum3/2
  height (m)/1 -> Sum3/1
  Sum3/1 -> proportional control gain/1
  proportional control gain/1 -> ref. velocity w (m/s)/1

== system ARDroneHover_2020b/Outer-loop Controller/Baseline Controller/Lateral velocity controller ==
  lateral velocity v (m/s) : Inport
  lateral velocity v ref. (m/s) : Inport  Port=2
  Gain1 : Gain  Gain=0.4
  Sum5 : Sum  Inputs=|-+
  roll angle ref. (rad) : Outport  VectorParamsAs1DForOutWhenUnconnected=off
  wires:
  lateral velocity v ref. (m/s)/1 -> Sum5/2
  Gain1/1 -> roll angle ref. (rad)/1
  Sum5/1 -> Gain1/1
  lateral velocity v (m/s)/1 -> Sum5/1

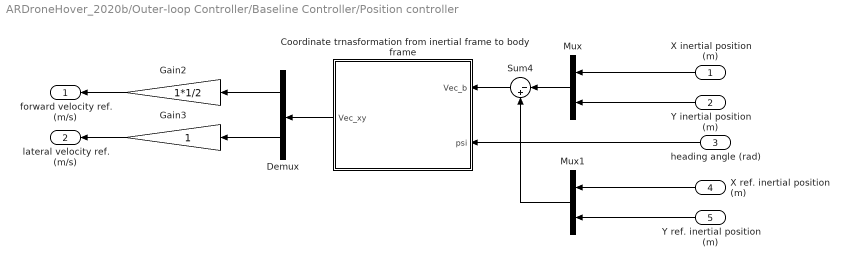
== system ARDroneHover_2020b/Outer-loop Controller/Baseline Controller/Position controller ==
  X inertial position (m) : Inport
  Y inertial position (m) : Inport  Port=2
  heading angle (rad) : Inport  Port=3
  X ref. inertial position (m) : Inport  Port=4
  Y ref. inertial position (m) : Inport  Port=5
  "Coordinate trnasformation from inertial frame to body frame " : MATLAB Function  TreatAsAtomicUnit=on
  Demux : Demux  Outputs=2
  Gain2 : Gain  Gain=1*1/2
  Gain3 : Gain
  Mux : Mux  Inputs=2
  Mux1 : Mux  Inputs=2
  Sum4 : Sum  Inputs=|-+
  forward velocity ref. (m/s) : Outport  VectorParamsAs1DForOutWhenUnconnected=off
  lateral velocity ref. (m/s) : Outport  Port=2  VectorParamsAs1DForOutWhenUnconnected=off
  wires:
  Gain3/1 -> lateral velocity ref. (m/s)/1
  Demux/2 -> Gain3/1
  Demux/1 -> Gain2/1
  Y ref. inertial position (m)/1 -> Mux1/2
  X ref. inertial position (m)/1 -> Mux1/1
  Mux/1 -> Sum4/1
  X inertial position (m)/1 -> Mux/1
  Y inertial position (m)/1 -> Mux/2
  Sum4/1 -> "Coordinate trnasformation from inertial frame to body frame "/1(Vec_b)
  Mux1/1 -> Sum4/2
  "Coordinate trnasformation from inertial frame to body frame "/1(Vec_xy) -> Demux/1
  heading angle (rad)/1 -> "Coordinate trnasformation from inertial frame to body frame "/2(psi)
  Gain2/1 -> forward velocity ref. (m/s)/1

== matlab function ARDroneHover_2020b/Data to States/Compute the Derivative/MATLAB Function ==
  data: u input; y output
function y = ZOH_nan(u)

persistent u_

if isempty(u_)
    u_ = 0;
end

if isnan(u)
    u = u_;
else
    u_ = u;
end

y = u;

== matlab function ARDroneHover_2020b/Data to States/Compute the Derivative/MATLAB Function1 ==
  data: u input; y output
function y = ZOH_nan(u)

persistent u_

if isempty(u_)
    u_ = 0;
end

if isnan(u)
    u = u_;
else
    u_ = u;
end

y = u;

== matlab function ARDroneHover_2020b/Data to States/Compute the Derivative/MATLAB Function2 ==
  data: u input; y output
function y = ZOH_nan(u)

persistent u_

if isempty(u_)
    u_ = 0;
end

if isnan(u)
    u = u_;
else
    u_ = u;
end

y = u;

== matlab function ARDroneHover_2020b/Data from Qualisys/Subsystem/MATLAB Function1 ==
  data: x4 output uint8; x3 output uint8; x2 output uint8; data input; x1 output uint8; object input
function [x4,x3,x2,x1] = fcn(data,object)

slot=(object-1)*8;

x1=data(41+slot);
x2=data(41+slot+1);
x3=data(41+slot+2);
x4=data(41+slot+3);

== matlab function ARDroneHover_2020b/Data from Qualisys/Subsystem/MATLAB Function2 ==
  data: x input uint32 size=1; X output single size=1; y input; Y output; z input; roll input; pitch input; yaw input; Z output; Roll output; Pitch output; Yaw output
function [X,Y,Z,Roll,Pitch,Yaw] = fcn(x,y,z,roll,pitch,yaw)


X = typecast(uint32(x),'single');
Y = typecast(uint32(y),'single');
Z = typecast(uint32(z),'single');
Roll = typecast(uint32(roll),'single');
Pitch = typecast(uint32(pitch),'single');
Yaw = typecast(uint32(yaw),'single');

== matlab function ARDroneHover_2020b/Data from Qualisys/Subsystem/MATLAB Function3 ==
  data: y4 output uint8; y3 output uint8; y2 output uint8; data input; y1 output uint8; object input
function [y4,y3,y2,y1] = fcn(data,object)

slot=(object-1)*8;

y1=data(45+slot);
y2=data(45+slot+1);
y3=data(45+slot+2);
y4=data(45+slot+3);

== matlab function ARDroneHover_2020b/Data from Qualisys/Subsystem/MATLAB Function4 ==
  data: z4 output uint8; z3 output uint8; z2 output uint8; data input; z1 output uint8; object input
function [z4,z3,z2,z1] = fcn(data,object)

slot=(object-1)*8;

z1=data(49+slot);
z2=data(49+slot+1);
z3=data(49+slot+2);
z4=data(49+slot+3);

== matlab function ARDroneHover_2020b/Data from Qualisys/Subsystem/MATLAB Function5 ==
  data: roll4 output uint8; roll3 output uint8; roll2 output uint8; data input; roll1 output uint8; object input
function [roll4,roll3,roll2,roll1] = fcn(data,object)

slot=(object-1)*8;

roll1=data(53+slot);
roll2=data(53+slot+1);
roll3=data(53+slot+2);
roll4=data(53+slot+3);

== matlab function ARDroneHover_2020b/Data from Qualisys/Subsystem/MATLAB Function6 ==
  data: pitch4 output uint8; pitch3 output uint8; pitch2 output uint8; data input; pitch1 output uint8; object input
function [pitch4,pitch3,pitch2,pitch1] = fcn(data,object)

slot=(object-1)*8;

pitch1=data(57+slot);
pitch2=data(57+slot+1);
pitch3=data(57+slot+2);
pitch4=data(57+slot+3);

== matlab function ARDroneHover_2020b/ARDrone Wi-Fi  Block/Subsystem1/Drone state request ==
  data: status input; fly input; rollAngRef input; pitchAngRef input; yawRateRef input; wRef input; enableRefs input; dataControl output; isFlying output; stop input; error output
function [dataControl, isFlying, error] = fcn( status, fly, rollAngRef, pitchAngRef, yawRateRef, wRef, enableRefs, stop)
%#codegen

% Persistent variables.
persistent SequenceNumber ;

% Initialization of persistent variables at first time step. 

if isempty(SequenceNumber)
    SequenceNumber = 1 ;
end



% Error code / No error: 0
error=0;

% Boolean of flying status / Flying: 1
isFlying = status(32) ;

% Byte array of size 150 to be sent to the drone.
strOut = uint8(zeros(150,1)) ;

% String that coontains a variable size command. 
% cmd is concatenated with previous commands at each sample
cmd = '';

% At first time step and every 100 time steps, data is requested.
if (SequenceNumber <=1 || mod(SequenceNumber, 100) ==0 )
    SequenceNumber = SequenceNumber+1; 
    strCmd = getString(SequenceNumber) ;
    cmd = ['AT*CONFIG=' strCmd ',"general:navdata_demo","TRUE"' char(13)];
    
end

SequenceNumber = SequenceNumber+1;
strCmd = getString(SequenceNumber) ;
cmd = [cmd 'AT*COMWDG=' strCmd char(13)];


if stop ==1 % Emergency stop
   cmd = ['AT*REF=' strCmd ',290717952' char(13)] ; 
    
else % Not emergency stop
    
    if SequenceNumber >20 && SequenceNumber <22
        
        % Trim vehicle state estimation / angles set to zero
        SequenceNumber =SequenceNumber+1;
        strCmd = getString(SequenceNumber) ;
        cmd = [cmd 'AT*FTRIM=' strCmd char(13)] ;
        
    elseif SequenceNumber >=22 && SequenceNumber <25
        cmd = [cmd 'AT*CONFIG=' strCmd '"conrol:altitude_max","100000"' char(13)] ;
        
        
    elseif SequenceNumber >=25
        
        if ( fly == 1  )
            
            if (isFlying ==0)
                
                SequenceNumber =SequenceNumber+1;
                strCmd = getString(SequenceNumber) ;
                cmd = [cmd 'AT*REF=' strCmd ',290718208' char(13)] ;
            
            elseif isFlying==1 && enableRefs==1
                
                SequenceNumber =SequenceNumber+1;
                strCmd = getString(SequenceNumber) ;
                      
                cmd = [cmd 'AT*PCMD=' strCmd ',1,'] ;
                 
                aux = double (float2IEEE754 (rollAngRef) )  ;
                strAux = getString(abs(aux)) ; 
                if rollAngRef<0
                   strAux = [char(45) strAux] ; 
                end
                cmd = [cmd strAux ','];
                      
               aux = double (float2IEEE754 (pitchAngRef) ) ;
               strAux = getString(abs(aux)) ; 
               if pitchAngRef<0
                    strAux = [char(45) strAux] ; 
               end
               cmd = [cmd strAux ','];
                      
               aux =  double(float2IEEE754 (wRef)) ;
               strAux = getString(abs(aux)) ; 
               if wRef<0
                    strAux = [char(45) strAux] ; 
               end
               cmd = [cmd strAux ','];
                      
                      
               aux =  double (float2IEEE754 (yawRateRef) ) ;
               strAux = getString(abs(aux)) ; 
               if yawRateRef <0
                     error=2; 
                     strAux = [char(45) strAux] ; 
               end
               cmd = [cmd strAux char(13)];
               
                
            end
            
            
        elseif ( fly==0 )
                
               if isFlying ==1
                    SequenceNumber =SequenceNumber+1;
                    strCmd = getString(SequenceNumber) ;
                    cmd = [cmd 'AT*REF=' strCmd ',290717696' char(13)] ;
                    
               end
        end
        
    end
    
    
    
end

% cmd must contain less than 150 bytes. 
if (length(cmd)<150)
    strOut(1:length(cmd)) = cmd ;
else
    error =1; 
end

dataControl = strOut;

end


%% My str2num function that allows for code generation
function [ strOut] = getString( a )
d=1;

if (a<10)
    d=1;
end

if (a >=10 && a <100)
    d=2;
end

if (a >=100 && a <1000)
    d=3;
end

if (a >=1000 && a <10000)
    d=4;
end

if (a >=10000 && a <100000)
    d=5;
end

if (a >=100000 && a <1000000)
    d=6;
end

if (a >=1000000 && a <10000000)
    d=7;
end

if (a >=10000000 && a <100000000)
    d=8;
end

if (a >=100000000 && a <1000000000)
    d=9;
end

if (a >=1000000000 && a <10000000000)
    d=10;
end

if (a >=10000000000 )
    d=11;
end



digit = uint8(zeros(1,d)) ;
resTotal = 0;
%d = length(a) ;
for k=1:d
    
    res1 = mod(a,10^k)/(10^(k-1)) ;
    %( mod(a,10*k) - resTotal)/(10*k) ;
    
    digit(d-k+1) = char(48 + res1);
    resTotal = (10^(k-1))*res1 +resTotal;
    
end

strOut = char(digit) ;


end

%% Function to obtain a IEEE754 representation of a float number
function [ iVal ] = float2IEEE754( fVal )

binData = dec2bin(typecast (single(fVal), 'uint8'),8) 

binData2 =[ binData(4,:) binData(3,:) binData(2,:) binData(1,:)] 
iVal =0; 
for k=32:-1:1
    
    if (binData2(k) =='1')
        bit = 1;
    else
        bit =0;
    end
    
    if k == 1
        iVal = iVal - bit*2^(31);
    else
        iVal = iVal + bit*2^(32-k) ; 
    end
    
end

iVal = int32(iVal)

end

== matlab function ARDroneHover_2020b/Data from Qualisys/Subsystem/MATLAB Function7 ==
  data: yaw4 output uint8; yaw3 output uint8; yaw2 output uint8; data input; yaw1 output uint8; object input
function [yaw4,yaw3,yaw2,yaw1] = fcn(data,object)

slot=(object-1)*8;

yaw1=data(61+slot);
yaw2=data(61+slot+1);
yaw3=data(61+slot+2);
yaw4=data(61+slot+3);

== matlab function ARDroneHover_2020b/Data to States/MATLAB Function ==
  data: v input; v_b output; phi input; theta input; psi input
function v_b = fcn(v,phi,theta,psi)

R = [cos(theta)*cos(psi)...
      sin(phi)*sin(theta)*cos(psi)-cos(phi)*sin(psi)...
      cos(phi)*sin(theta)*cos(psi)+sin(phi)*sin(psi);
   cos(theta)*sin(psi)...
   sin(phi)*sin(theta)*sin(psi)+cos(phi)*cos(psi)... 
   cos(phi)*sin(theta)*sin(psi)-sin(phi)*cos(psi);
   -sin(theta)...
   sin(phi)*cos(theta)...
   cos(phi)*cos(theta)];

v_b = R'*v;

== matlab function ARDroneHover_2020b/MATLAB Function1 ==
  data: on_off input; states input; t input; pd output; dot_pd output; ddot_pd output; psi_d output
function [pd, dot_pd, ddot_pd, psi_d] = desired_trajectory(on_off,states,t)
%#codegen

% ------------------------------------------------------------------------
% inputs:
% on_off - 1 if tracking is on, 0 if it is off
% states - structure with state variables
% t - current simulation time
% 
% outputs:
% pd - desired position
% dot_pd - desired velocity
% ddot_pd - desired acceleration
% psi_d - desired yaw angle
% ------------------------------------------------------------------------

persistent t0
persistent p0
persistent previous_status

on = 1;
off = 0;

if isempty(previous_status)
    previous_status = on;
    p0 = [states(7:8);-1];
end

if on_off == off
    if previous_status == on 
    % first time off or switching back off
        p0 = [states(7:8);-1]; % x0 and y0 match the current position
    end
    pd = p0;
    dot_pd = [0;0;0];
    ddot_pd = [0;0;0];
    psi_d = 0;
else
    if isempty(t0) || (previous_status == off) 
    % first time on or switching back on
        t0 = t;
        p0 = [states(7:8);-1];
    end
    dt = t-t0;

%!!!!!!!!!!!!!!!!!!!!!!!!!!!!!!!!!!!!!!!!!!!!!!!!!!!!!!!!!!!!!!!!!!!!!!!!
% replace with the necessary code to define adequate desired trajectories
% use dt, p0, and any additional parameters
%     pd = p0;
%     dot_pd = [0;0;0];
%     ddot_pd = [0;0;0];
%     psi_d = 0;
% 
    om = 0.5;
    pd = p0 + [cos(om*dt)-1;sin(om*dt);0];%[0.5*dt;0;0];
    dot_pd = om*[-sin(om*dt);cos(om*dt);0];%[0.5;0;0];
    ddot_pd = om^2*[-cos(om*dt);-sin(om*dt);0];%[0;0;0];
    psi_d = om*dt;

%     pd = p0 + [0.5*dt;0;0];
%     dot_pd = [0.5;0;0];
%     ddot_pd = [0;0;0];
%     psi_d = 0;
%     
%     if pd(1) > 1
%         pd(1) = 1;
%         dot_pd(1) = 0;
%     end
    
%     Delta = 0.5;
%     V = 1;
%     psi_d = atan2(-(states(8)-1),Delta);
%     dot_psi_d = -states(5)/Delta/(1+((states(8)-1)/Delta)^2);
%     dot_pd = V*[cos(psi_d);sin(psi_d);0];
%     ddot_pd = V*dot_psi_d*[-sin(psi_d);cos(psi_d);0];
%     pd = [states(7:8);-1];
%     psi_d = 0;

%!!!!!!!!!!!!!!!!!!!!!!!!!!!!!!!!!!!!!!!!!!!!!!!!!!!!!!!!!!!!!!!!!!!!!!!!

end

previous_status = on_off;
